simulink model "mod_sim_VTMS"  (R2018b)
settings: Solver=FixedStepDiscrete  StartTime=0.0  StopTime=t_Simulation  FixedStep=delta_t  RelTol=1e-3
values from neighbouring files (symbols this model uses):
  P_charge = 150    [main_sim_VTMS.m]
undefined symbols (not defined in the file or in its folder): A_EMaschine_Getriebe, A_j_c, A_Stirn, Anzahl_Peltierelemente, b_Batteriepack, b_c, b_EMaschine, b_Getriebe, b_j, b_Ladegeraet, BatPara, c_W, delta_t, DiscIntNeverNeededParam, e_Fahrzeug, eta_EMaschine_Break_M_EMaschine, eta_EMaschine_Break_n_EMaschine, eta_EMaschine_Faktor_Volllast, eta_EMaschine_Table, eta_Getriebe, eta_Ladegeraet, eta_Leistungselektronik_Break_M_EMaschine, eta_Leistungselektronik_Break_n_EMaschine, eta_Leistungselektronik_Faktor_Volllast, eta_Leistungselektronik_Table, f_R, I_DT_U_Break_DT, I_DT_U_Break_U, I_DT_U_Value_I, i_Getriebe, I_max, Ladevorgang, M_EMaschine_max, m_Fahrzeug, m_Zuladung, n_Zelle, P_Nebenverbraucher, p_Zelle, Peltier_Max_Eff, Q_DT_U_Break_DT, Q_DT_U_Break_U, Q_DT_U_Value_Q, Q_Imax_DT_Break_DT, Q_Imax_DT_Value_Q, r_dynamisch, rho_Luft, s_Zelle, SOC_init, Steuerung_Kuehlerluefter, Steuerung_Pumpe, Steuerung_Ventil, switch_BP_Zyklus, T_Batteriepack_init, T_EMaschine_Getriebe_init, T_Ladegeraet_init, T_Ladegeraet_Offset, T_Leistungselektronik_init, T_Offset_Batteriepack, T_Offset_EMaschine_Getriebe, T_Offset_Leistungselektronik ... (+36)
libraries: simulink x3, simulink_extras x2
(part 1 of 5)
settings Model: SimulationMode=accelerator  NumberOfSteps=100  Creator=Hannes  LastModifiedBy=gu74niw
settings SolverCC: InsertRTBMode=Always
settings DataIOCC: SaveOutput=off  SignalLogging=off  DSMLogging=off  SaveTime=off
settings OptimizationCC: DefaultParameterBehavior=Inlined  UseDivisionForNetSlopeComputation=on  PassReuseOutputArgsAs=Individual arguments  EfficientFloat2IntCast=on  EfficientMapNaN2IntZero=off  MaxStackSize=inf  SimCompilerOptimization=on
settings DebuggingCC: ReadBeforeWriteMsg=DisableAll  WriteAfterWriteMsg=DisableAll  WriteAfterReadMsg=DisableAll  AlgebraicLoopMsg=error  MultiTaskDSMMsg=none  IntegerOverflowMsg=error  ParameterUnderflowMsg=error  ParameterTunabilityLossMsg=error  AssertControl=DisableAll  AllowSymbolicDim=off  StrictBusMsg=ErrorOnBusTreatedAsVector  NonBusSignalsTreatedAsBus=error  SFInvalidInputDataAccessInChartInitDiag=error  SFTransitionOutsideNaturalParentDiag=error  SFUnreachableExecutionPathDiag=error  SFUndirectedBroadcastEventsDiag=error  SFTransitionActionBeforeConditionDiag=error  IntegerSaturationMsg=error
settings ModelReferenceCC: UpdateModelReferenceTargets=IfOutOfDate
settings SFSimCC: SFSimEcho=off  SimUseLocalCustomCode=off  MATLABDynamicMemAlloc=off
settings RTWCC: SystemTargetFile=ert.tlc  TemplateMakefile=RTW.MSVCBuild  Description=Create Visual C/C++ Solution File for Embedded Coder  GenerateReport=on  RTWUseLocalCustomCode=off  IncludeHyperlinkInReport=on  LaunchReport=on  GenerateTraceInfo=on  GenerateTraceReport=on  GenerateTraceReportSl=on  GenerateTraceReportSf=on  GenerateTraceReportEml=on
settings CodeAppCC: ForceParamTrailComments=on  IgnoreCustomStorageClasses=off  OperatorAnnotations=on  SimulinkDataObjDesc=on  SFDataObjDesc=on  InsertBlockDesc=on
settings ERTTargetCC: TargetLangStandard=C99 (ISO)  GenerateSampleERTMain=on  InlinedParameterPlacement=NonHierarchical  ERTCustomFileTemplate=example_file_process.tlc
settings ConfigComp: CovScope=ReferencedModels  CovIncludeTopModel=off

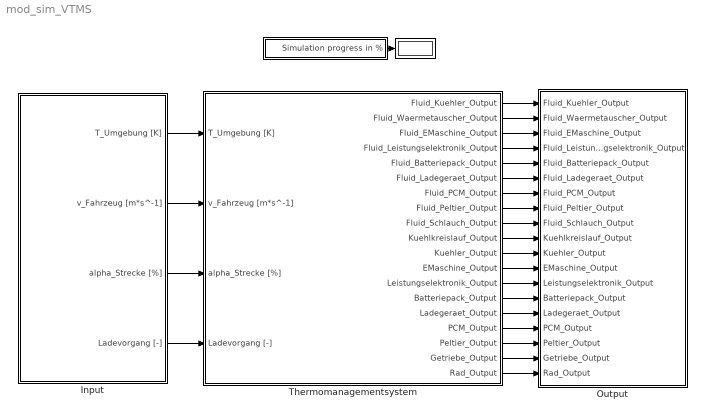
== system mod_sim_VTMS ==
  "\t\t     " : Subsystem
  " " : Display
      settings: Format=bank
  Input : Subsystem
  Output : Subsystem
  Thermomanagementsystem : Subsystem
  wires:
  "\t\t     "/1(Simulation progress in %) -> " "/1
  Input/1(T_Umgebung [K]) -> Thermomanagementsystem/1(T_Umgebung [K])
  Input/2(v_Fahrzeug [m*s^-1]) -> Thermomanagementsystem/2(v_Fahrzeug [m*s^-1])
  Input/3(alpha_Strecke [%]) -> Thermomanagementsystem/3(alpha_Strecke [%])
  Input/4(Ladevorgang [-]) -> Thermomanagementsystem/4(Ladevorgang [-])
  Thermomanagementsystem/1(Fluid_Kuehler_Output) -> Output/1(Fluid_Kuehler_Output)
  Thermomanagementsystem/2(Fluid_Waermetauscher_Output) -> Output/2(Fluid_Waermetauscher_Output)
  Thermomanagementsystem/3(Fluid_EMaschine_Output) -> Output/3(Fluid_EMaschine_Output)
  Thermomanagementsystem/4(Fluid_Leistungselektronik_Output) -> Output/4(Fluid_Leistungselektronik_Output)
  Thermomanagementsystem/5(Fluid_Batteriepack_Output) -> Output/5(Fluid_Batteriepack_Output)
  Thermomanagementsystem/6(Fluid_Ladegeraet_Output) -> Output/6(Fluid_Ladegeraet_Output)
  Thermomanagementsystem/7(Fluid_PCM_Output) -> Output/7(Fluid_PCM_Output)
  Thermomanagementsystem/8(Fluid_Peltier_Output) -> Output/8(Fluid_Peltier_Output)
  Thermomanagementsystem/9(Fluid_Schlauch_Output) -> Output/9(Fluid_Schlauch_Output)
  Thermomanagementsystem/10(Kuehlkreislauf_Output) -> Output/10(Kuehlkreislauf_Output)
  Thermomanagementsystem/11(Kuehler_Output) -> Output/11(Kuehler_Output)
  Thermomanagementsystem/12(EMaschine_Output) -> Output/12(EMaschine_Output)
  Thermomanagementsystem/13(Leistungselektronik_Output) -> Output/13(Leistungselektronik_Output)
  Thermomanagementsystem/14(Batteriepack_Output) -> Output/14(Batteriepack_Output)
  Thermomanagementsystem/15(Ladegeraet_Output) -> Output/15(Ladegeraet_Output)
  Thermomanagementsystem/16(PCM_Output) -> Output/16(PCM_Output)
  Thermomanagementsystem/17(Peltier_Output) -> Output/17(Peltier_Output)
  Thermomanagementsystem/18(Getriebe_Output) -> Output/18(Getriebe_Output)
  Thermomanagementsystem/19(Rad_Output) -> Output/19(Rad_Output)

== system mod_sim_VTMS/		      ==
  note: Fortschritt der Simulation = 100 * simulierte Zeit / t_Simulation
      |
      | mit Fortschritt der Simulation in %
  Clock : Clock
  Constant : Constant  Value=t_Simulation  VectorParams1D=off
  Divide : Product  Inputs=*/
  Umrechnung in % : Gain  Gain=100
  Simulation progress in % : Outport
  wires:
  Constant/1 -> Divide/2
  Clock/1 -> Divide/1
  Divide/1 -> Umrechnung in %/1
  Umrechnung in %/1 -> Simulation progress in %/1

== system mod_sim_VTMS/Input ==
  note: Umrechnung km/h in m/s
  note: Nur positive Geschwindigkeit
  Constant : Constant  Value=T_Umgebung
  Constant1 : Constant  Commented=on  Value=Ladevorgang
  Data Type Conversion : DataTypeConversion  OutDataTypeStr=boolean
  From Workspace : FromWorkspace  VariableName=v_Fahrzeug  SampleTime=0  OutputAfterFinalValue=Setting to zero
  From Workspace1 : FromWorkspace  VariableName=alpha_Strecke  SampleTime=0  OutputAfterFinalValue=Setting to zero
  From Workspace2 : FromWorkspace  VariableName=Ladevorgang  SampleTime=0  OutputAfterFinalValue=Setting to zero
  Gain : Gain  Gain=1/3.6
  Saturation : Saturate  UpperLimit=inf  LowerLimit=0
  T_Umgebung [K] : Outport
  v_Fahrzeug [m*s^-1] : Outport  Port=2
  alpha_Strecke [%] : Outport  Port=3
  Ladevorgang [-] : Outport  Port=4
  wires:
  Constant/1 -> T_Umgebung [K]/1
  Saturation/1 -> Gain/1
  From Workspace/1 -> Saturation/1
  Gain/1 -> v_Fahrzeug [m*s^-1]/1
  From Workspace1/1 -> alpha_Strecke [%]/1
  From Workspace2/1 -> Data Type Conversion/1
  Data Type Conversion/1 -> Ladevorgang [-]/1

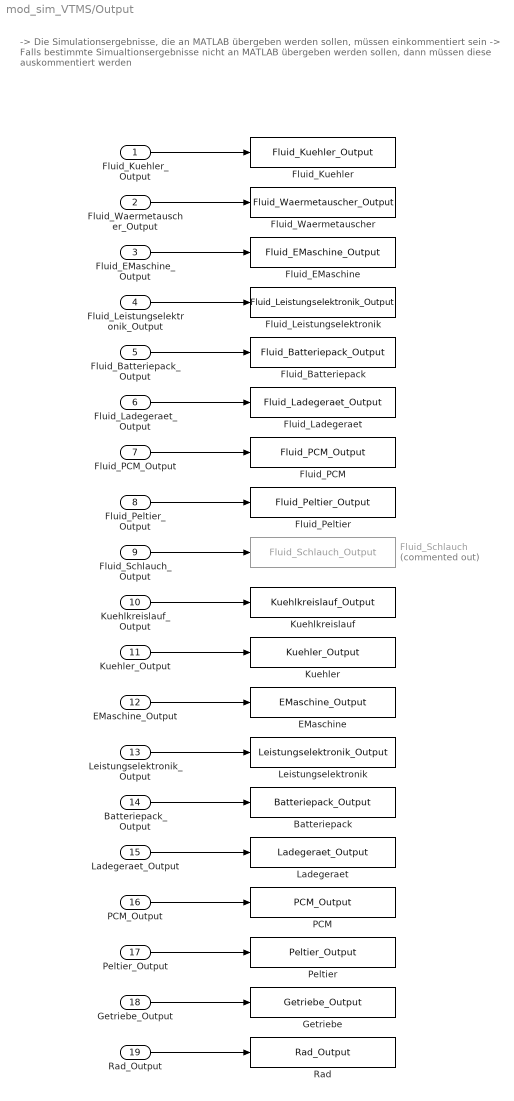
== system mod_sim_VTMS/Output ==
  note: -> Die Simulationsergebnisse, die an MATLAB übergeben werden sollen, müssen einkommentiert sein
      | -> Falls bestimmte Simualtionsergebnisse nicht an MATLAB übergeben werden sollen, dann müssen diese auskommentiert werden
  Fluid_Kuehler_Output : Inport
  Fluid_Waermetauscher_Output : Inport  Port=2
  Fluid_EMaschine_Output : Inport  Port=3
  Fluid_Leistungselektronik_Output : Inport  Port=4
  Fluid_Batteriepack_Output : Inport  Port=5
  Fluid_Ladegeraet_Output : Inport  Port=6
  Fluid_PCM_Output : Inport  Port=7
  Fluid_Peltier_Output : Inport  Port=8
  Fluid_Schlauch_Output : Inport  Port=9
  Kuehlkreislauf_Output : Inport  Port=10
  Kuehler_Output : Inport  Port=11
  EMaschine_Output : Inport  Port=12
  Leistungselektronik_Output : Inport  Port=13
  Batteriepack_Output : Inport  Port=14
  Ladegeraet_Output : Inport  Port=15
  PCM_Output : Inport  Port=16
  Peltier_Output : Inport  Port=17
  Getriebe_Output : Inport  Port=18
  Rad_Output : Inport  Port=19
  Batteriepack : ToWorkspace  VariableName=Batteriepack_Output  SaveFormat=Timeseries  SampleTime=-1
      settings: Decimation=Decimation_Output
  EMaschine : ToWorkspace  VariableName=EMaschine_Output  SaveFormat=Timeseries  SampleTime=-1
      settings: Decimation=Decimation_Output
  Fluid_Batteriepack : ToWorkspace  VariableName=Fluid_Batteriepack_Output  SaveFormat=Timeseries  SampleTime=-1
      settings: Decimation=Decimation_Output
  Fluid_EMaschine : ToWorkspace  VariableName=Fluid_EMaschine_Output  SaveFormat=Timeseries  SampleTime=-1
      settings: Decimation=Decimation_Output
  Fluid_Kuehler : ToWorkspace  VariableName=Fluid_Kuehler_Output  SaveFormat=Timeseries  SampleTime=-1
      settings: Decimation=Decimation_Output
  Fluid_Ladegeraet : ToWorkspace  VariableName=Fluid_Ladegeraet_Output  SaveFormat=Timeseries  SampleTime=-1
      settings: Decimation=Decimation_Output
  Fluid_Leistungselektronik : ToWorkspace  VariableName=Fluid_Leistungselektronik_Output  SaveFormat=Timeseries  SampleTime=-1
      settings: Decimation=Decimation_Output
  Fluid_PCM : ToWorkspace  VariableName=Fluid_PCM_Output  SaveFormat=Timeseries  SampleTime=-1
      settings: Decimation=Decimation_Output
  Fluid_Peltier : ToWorkspace  VariableName=Fluid_Peltier_Output  SaveFormat=Timeseries  SampleTime=-1
      settings: Decimation=Decimation_Output
  Fluid_Schlauch : ToWorkspace  Commented=on  VariableName=Fluid_Schlauch_Output  SaveFormat=Timeseries  SampleTime=-1
      settings: Decimation=Decimation_Output
  Fluid_Waermetauscher : ToWorkspace  VariableName=Fluid_Waermetauscher_Output  SaveFormat=Timeseries  SampleTime=-1
      settings: Decimation=Decimation_Output
  Getriebe : ToWorkspace  VariableName=Getriebe_Output  SaveFormat=Timeseries  SampleTime=-1
      settings: Decimation=Decimation_Output
  Kuehler : ToWorkspace  VariableName=Kuehler_Output  SaveFormat=Timeseries  SampleTime=-1
      settings: Decimation=Decimation_Output
  Kuehlkreislauf : ToWorkspace  VariableName=Kuehlkreislauf_Output  SaveFormat=Timeseries  SampleTime=-1
      settings: Decimation=Decimation_Output
  Ladegeraet : ToWorkspace  VariableName=Ladegeraet_Output  SaveFormat=Timeseries  SampleTime=-1
      settings: Decimation=Decimation_Output
  Leistungselektronik : ToWorkspace  VariableName=Leistungselektronik_Output  SaveFormat=Timeseries  SampleTime=-1
      settings: Decimation=Decimation_Output
  PCM : ToWorkspace  VariableName=PCM_Output  SaveFormat=Timeseries  SampleTime=-1
      settings: Decimation=Decimation_Output
  Peltier : ToWorkspace  VariableName=Peltier_Output  SaveFormat=Timeseries  SampleTime=-1
      settings: Decimation=Decimation_Output
  Rad : ToWorkspace  VariableName=Rad_Output  SaveFormat=Timeseries  SampleTime=-1
      settings: Decimation=Decimation_Output
  wires:
  Ladegeraet_Output/1 -> Ladegeraet/1
  Fluid_Ladegeraet_Output/1 -> Fluid_Ladegeraet/1
  PCM_Output/1 -> PCM/1
  Kuehler_Output/1 -> Kuehler/1
  Kuehlkreislauf_Output/1 -> Kuehlkreislauf/1
  Fluid_PCM_Output/1 -> Fluid_PCM/1
  Fluid_Kuehler_Output/1 -> Fluid_Kuehler/1
  Fluid_EMaschine_Output/1 -> Fluid_EMaschine/1
  Leistungselektronik_Output/1 -> Leistungselektronik/1
  Rad_Output/1 -> Rad/1
  Fluid_Schlauch_Output/1 -> Fluid_Schlauch/1
  Fluid_Peltier_Output/1 -> Fluid_Peltier/1
  EMaschine_Output/1 -> EMaschine/1
  Fluid_Batteriepack_Output/1 -> Fluid_Batteriepack/1
  Fluid_Leistungselektronik_Output/1 -> Fluid_Leistungselektronik/1
  Batteriepack_Output/1 -> Batteriepack/1
  Getriebe_Output/1 -> Getriebe/1
  Peltier_Output/1 -> Peltier/1
  Fluid_Waermetauscher_Output/1 -> Fluid_Waermetauscher/1

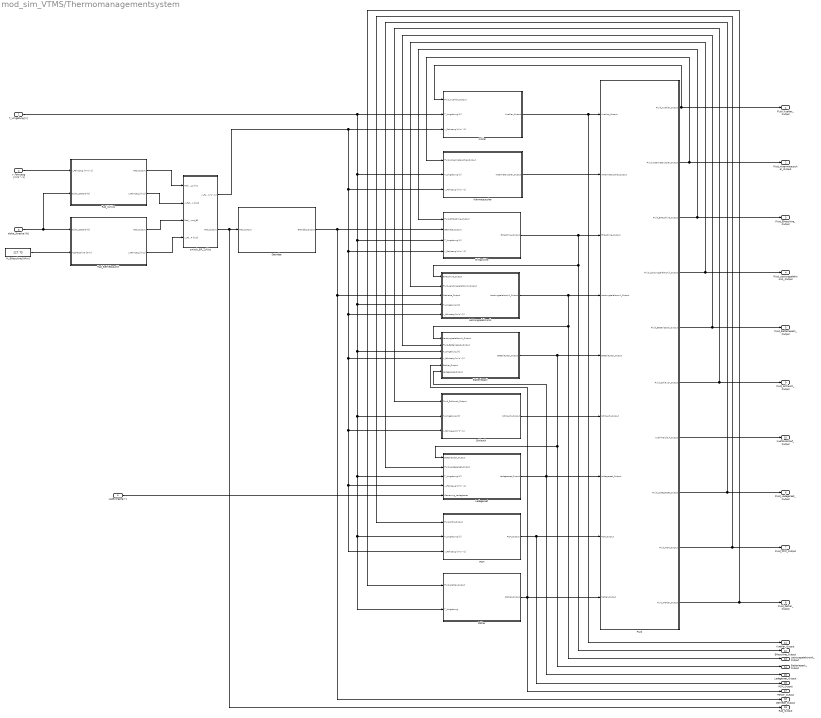
== system mod_sim_VTMS/Thermomanagementsystem ==
  T_Umgebung [K] : Inport
  v_Fahrzeug [m*s^-1] : Inport  Port=2
  alpha_Strecke [%] : Inport  Port=3
  Ladevorgang [-] : Inport  Port=4
  Batteriepack : Subsystem
  E-Maschine : Subsystem
  Fluid : Subsystem
  Getriebe : Subsystem
  Kühler : Subsystem
  Ladegeraet : Subsystem
  Leistungselektronik : Subsystem
  M_EMaschine [N*m] : Constant  Value=127.75
  PCM : Subsystem
  Peltier : Subsystem
  Rad_Betriebspunkt : Subsystem
  Rad_Zyklus : Subsystem
  Schlauch : Subsystem
  Wärmetauscher : Subsystem
  switch_BP_Zyklus : Subsystem
  Fluid_Kuehler_Output : Outport
  Fluid_Waermetauscher_Output : Outport  Port=2
  Fluid_EMaschine_Output : Outport  Port=3
  Fluid_Leistungselektronik_Output : Outport  Port=4
  Fluid_Batteriepack_Output : Outport  Port=5
  Fluid_Ladegeraet_Output : Outport  Port=6
  Fluid_PCM_Output : Outport  Port=7
  Fluid_Peltier_Output : Outport  Port=8
  Fluid_Schlauch_Output : Outport  Port=9
  Kuehlkreislauf_Output : Outport  Port=10
  Kuehler_Output : Outport  Port=11
  EMaschine_Output : Outport  Port=12
  Leistungselektronik_Output : Outport  Port=13
  Batteriepack_Output : Outport  Port=14
  Ladegeraet_Output : Outport  Port=15
  PCM_Output : Outport  Port=16
  Peltier_Output : Outport  Port=17
  Getriebe_Output : Outport  Port=18
  Rad_Output : Outport  Port=19
  wires:
  alpha_Strecke [%]/1 -> Rad_Zyklus/2(alpha_Strecke [%]), Rad_Betriebspunkt/1(alpha_Strecke [%])
  Getriebe/1(Getriebe_Output) -> E-Maschine/2(Getriebe_Output), Getriebe_Output/1, Leistungselektronik/3(Getriebe_Output)
  E-Maschine/1(EMaschine_Output) -> Leistungselektronik/1(EMaschine_Output), EMaschine_Output/1, Fluid/3(EMaschine_Output)
  Leistungselektronik/1(Leistungselektronik_Output) -> Batteriepack/1(Leistungselektronik_Output), Leistungselektronik_Output/1, Fluid/4(Leistungselektronik_Output)
  Batteriepack/1(Batteriepack_Output) -> Fluid/5(Batteriepack_Output), Ladegeraet/1(Batteriepack_Output), Batteriepack_Output/1
  Fluid/6(Fluid_Schlauch_Output) -> Fluid_Schlauch_Output/1, Schlauch/1(Fluid_Schlauch_Output)
  Wärmetauscher/1(Waermetauscher_Output) -> Fluid/2(Waermetauscher_Output)
  T_Umgebung [K]/1 -> Kühler/2(T_Umgebung [K]), Ladegeraet/3(T_Umgebung [K]), Peltier/2(T_Umgebung), PCM/2(T_Umgebung [K]), Schlauch/2(T_Umgebung [K]), Batteriepack/3(T_Umgebung [K]), Leistungselektronik/4(T_Umgebung [K]), E-Maschine/3(T_Umgebung [K]), Wärmetauscher/2(T_Umgebung [K])
  Kühler/1(Kuehler_Output) -> Kuehler_Output/1, Fluid/1(Kuehler_Output)
  Fluid/2(Fluid_Waermetauscher_Output) -> Fluid_Waermetauscher_Output/1, Wärmetauscher/1(Fluid_Waermetauscher_Output)
  Fluid/4(Fluid_Leistungselektronik_Output) -> Fluid_Leistungselektronik_Output/1, Leistungselektronik/2(Fluid_Leistungselektronik_Output)
  Fluid/5(Fluid_Batteriepack_Output) -> Fluid_Batteriepack_Output/1, Batteriepack/2(Fluid_Batteriepack_Output)
  Schlauch/1(Schlauch_Output) -> Fluid/6(Schlauch_Output)
  Fluid/1(Fluid_Kuehler_Output) -> Fluid_Kuehler_Output/1, Kühler/1(Fluid_Kuehler_Output)
  Fluid/3(Fluid_EMaschine_Output) -> Fluid_EMaschine_Output/1, E-Maschine/1(Fluid_EMaschine_Output)
  Fluid/7(Kuehlkreislauf_Output) -> Kuehlkreislauf_Output/1
  Ladegeraet/1(Ladegeraet_Output) -> Ladegeraet_Output/1, Batteriepack/6(Ladegeraet_Output), Fluid/7(Ladegeraet_Output)
  PCM/1(PCM_Output) -> PCM_Output/1, Fluid/8(PCM_Output)
  Ladevorgang [-]/1 -> Ladegeraet/5(Steuerung_Ladegeraet)
  Peltier/1(Peltier_Output) -> Peltier_Output/1, Batteriepack/5(Peltier_Output), Fluid/9(Peltier_Output)
  Fluid/8(Fluid_Ladegeraet_Output) -> Ladegeraet/2(Fluid_Ladegeraet_Output), Fluid_Ladegeraet_Output/1
  Fluid/9(Fluid_PCM_Output) -> Fluid_PCM_Output/1, PCM/1(Fluid_PCM_Output)
  Fluid/10(Fluid_Peltier_Output) -> Peltier/1(Fluid_Peltier_Output), Fluid_Peltier_Output/1
  M_EMaschine [N*m]/1 -> Rad_Betriebspunkt/2(M_EMaschine [N*m])
  v_Fahrzeug [m*s^-1]/1 -> Rad_Zyklus/1(v_Fahrzeug [m*s^-1])
  switch_BP_Zyklus/1(v_Fahrzeug [m*s^-1]) -> Kühler/3(v_Fahrzeug [m*s^-1]), Ladegeraet/4(v_Fahrzeug [m*s^-1]), PCM/3(v_Fahrzeug [m*s^-1]), Schlauch/3(v_Fahrzeug [m*s^-1]), Batteriepack/4(v_Fahrzeug [m*s^-1]), Leistungselektronik/5(v_Fahrzeug [m*s^-1]), E-Maschine/4(v_Fahrzeug [m*s^-1]), Wärmetauscher/3(v_Fahrzeug [m*s^-1])
  switch_BP_Zyklus/2(Rad_Output) -> Rad_Output/1, Getriebe/1(Rad_Output)
  Rad_Zyklus/1(Rad_Output) -> switch_BP_Zyklus/1(Rad_Output_Zyklus)
  Rad_Zyklus/2(v_Fahrzeug [m/s]) -> switch_BP_Zyklus/2(v_Fahrzeug_Zyklus [m/s])
  Rad_Betriebspunkt/1(Rad_Output) -> switch_BP_Zyklus/3(Rad_Output_BP)
  Rad_Betriebspunkt/2(v_Fahrzeug [m/s]) -> switch_BP_Zyklus/4(v_Fahrzeug_BP [m/s])

== system mod_sim_VTMS/Thermomanagementsystem/Batteriepack ==
  note: Neben der Leistungsanforderung aus dem Fahrbetrieb belasten Nebenverbraucher des Fahrzeugs das Batteriepack
  Leistungselektronik_Output : Inport
  Fluid_Batteriepack_Output : Inport  Port=2
  T_Umgebung [K] : Inport  Port=3
  v_Fahrzeug [m*s^-1] : Inport  Port=4
  Peltier_Output : Inport  Port=5
  Ladegeraet_Output : Inport  Port=6
  "Abbruch, wenn SOC <= 0" : Subsystem
  Add : Sum  Inputs=++-+
  Batteriepack(1) elektrisch : Subsystem
  Batteriepack(1) thermisch : Subsystem
  Bus Creator : BusCreator  Inputs=6
  Bus Selector : BusSelector  OutputSignals=T_FinitesVolumen_Batteriepack(1) [K],PV_Kuehlfluessigkeit_Batteriepack(1) [m^3*s^-1]
  Bus Selector1 : BusSelector  OutputSignals=P_Batteriepack_Fahrbetrieb [W]
  Bus Selector2 : BusSelector  OutputSignals=P_Ladegeraet_Bat [W]
  Bus Selector3 : BusSelector  OutputSignals=P_Peltier_Bat [W]
  Constant : Constant  Value=P_Nebenverbraucher  VectorParams1D=off
  Batteriepack_Output : Outport
  wires:
  Bus Creator/1 -> Batteriepack_Output/1
  Batteriepack(1) elektrisch/5(P_Verlust_Batteriepack [W]) -> Batteriepack(1) thermisch/1(P_Verlust_Batteriepack [W])
  T_Umgebung [K]/1 -> Batteriepack(1) thermisch/4(T_Umgebung [K])
  v_Fahrzeug [m*s^-1]/1 -> Batteriepack(1) thermisch/5(v_Fahrzeug [m*s^-1])
  Batteriepack(1) thermisch/1(T_Batteriepack [K]) -> Batteriepack(1) elektrisch/1(T_Batteriepack [K]), Bus Creator/5  "T_Batteriepack [K]"
  Batteriepack(1) elektrisch/4(eta_Batteriepack [%]) -> Bus Creator/4  "eta_Batteriepack [%]"
  Batteriepack(1) elektrisch/2(U_Batteriepack [V]) -> Bus Creator/2  "U_Batteriepack [V]"
  Batteriepack(1) elektrisch/1(I_Batteriepack [A]) -> Bus Creator/1  "I_Batteriepack [A]"
  Batteriepack(1) thermisch/2(PQ_Batteriepack_FinitesVolumen [W]) -> Bus Creator/6  "PQ_Batteriepack(1)_FinitesVolumen [W]"
  Batteriepack(1) elektrisch/3(SOC_Batteriepack [-]) -> "Abbruch, wenn SOC <= 0"/1(SOC_Batteriepack [-]), Bus Creator/3  "SOC_Batteriepack [-]"
  Fluid_Batteriepack_Output/1 -> Bus Selector/1
  Bus Selector/1 -> Batteriepack(1) thermisch/2(T_FinitesVolumen [K])  "<T_FinitesVolumen_Batteriepack(1) [K]>"
  Bus Selector/2 -> Batteriepack(1) thermisch/3(PV_Kuehlfluessigkeit [m^3*s^-1])  "<PV_Kuehlfluessigkeit_Batteriepack(1) [m^3*s^-1]>"
  Bus Selector3/1 -> Add/4  "<P_Peltier_Bat [W]>"
  Bus Selector2/1 -> Add/3  "<P_Ladegeraet_Bat [W]>"
  Ladegeraet_Output/1 -> Bus Selector2/1
  Bus Selector1/1 -> Add/1  "<P_Batteriepack_Fahrbetrieb [W]>"
  Constant/1 -> Add/2
  Add/1 -> Batteriepack(1) elektrisch/2(P_Batteriepack [W])
  Peltier_Output/1 -> Bus Selector3/1
  Leistungselektronik_Output/1 -> Bus Selector1/1

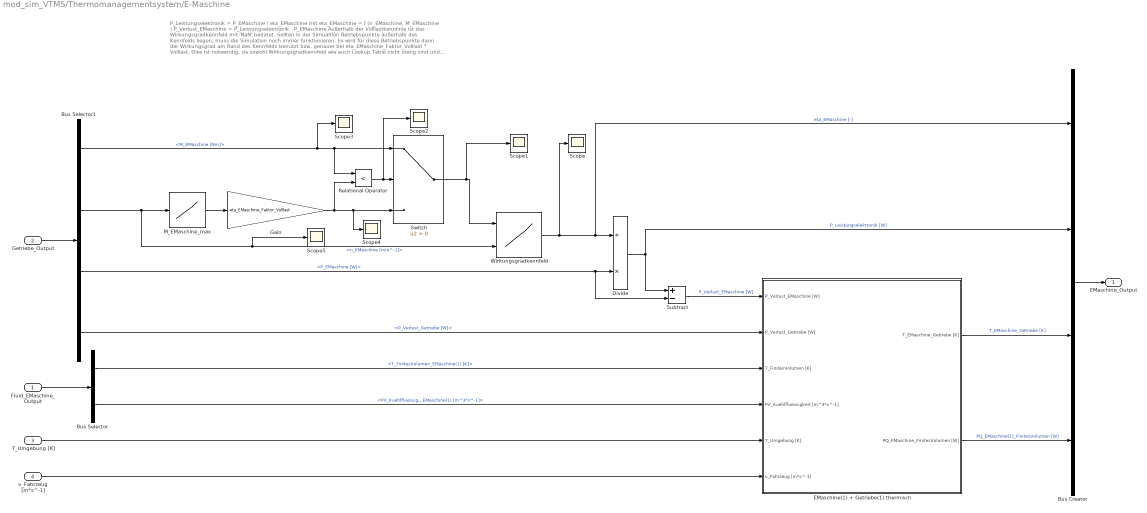
== system mod_sim_VTMS/Thermomanagementsystem/E-Maschine ==
  note: P_Leistungselektronik = P_EMaschine / eta_EMaschine
      |
      | mit eta_EMaschine = f (n_EMaschine, M_EMaschine )
      |
      | P_Verlust_EMaschine = P_Leistungselektronik - P_EMaschine
      |
      | Außerhalb der Volllastkennlinie ist das Wirkungsgradkennfeld mit 'NaN' bedatet. Sollten in der Simualtion Betriebspunkte außerhalb des Kennfelds liegen, muss die Simulation noch immer funktionieren. Es wird für diese Betriebspunkte dann der Wirkungsgrad am Rand des Kennfelds benutzt bzw. genauer bei eta_EMaschine_Faktor_Volllast * Volllast. Dies ist notwendig, da sowohl Wirkungsgradkennfeld wie auch Lookup Table nicht stetig sind und somit zwischen Stützstellen interpolieren müssen. Dies kann dazu führen, dass ein Wert, der auf der Volllastlinie sitzt, in 'NaN' im Wirkungsgradkennfeld resultiert. Um dies zu vermeiden, wird mit eta_EMaschine_Faktor_Volllast * Volllast gerechnet, wenn Betriebspunkte außerhalb des Kennfelds liegen, um 'NaN' Wirkungsgrade zu vermeiden. eta_EMaschine_Faktor_Volllast ist stark abh. von der Güte (Abstand der Stützstellen) des Wirkungsgradkennfeldes.
  Fluid_EMaschine_Output : Inport
  Getriebe_Output : Inport  Port=2
  T_Umgebung [K] : Inport  Port=3
  v_Fahrzeug [m*s^-1] : Inport  Port=4
  Bus Creator : BusCreator  Inputs=4
  Bus Selector : BusSelector  OutputSignals=T_FinitesVolumen_EMaschine(1) [K],PV_Kuehlfluessigkeit_EMaschine(1) [m^3*s^-1]
  Bus Selector1 : BusSelector  OutputSignals=M_EMaschine [Nm],n_EMaschine [min^-1],P_EMaschine [W],P_Verlust_Getriebe [W]
  Divide : Product  Inputs=/*
  EMaschine(1) + Getriebe(1) thermisch : Subsystem
  Gain : Gain  Gain=eta_EMaschine_Faktor_Volllast
  M_EMaschine_max : Lookup_n-D  NumberOfTableDimensions=1  BreakpointsForDimension1=M_EMaschine_max(1,:)  BeginIndexSearchUsingPreviousIndexResult=on  Table=M_EMaschine_max(2,:)  ExtrapMethod=Clip  UseLastTableValue=on  InternalRulePriority=Speed  RndMeth=Simplest  InputSameDT=on
  Relational Operator : RelationalOperator  Operator=<  OutDataTypeStr=boolean  RndMeth=Simplest
  Scope{,1..5} (6 alike) : Scope
  Subtract : Sum  Inputs=+-
  Switch : Switch  Criteria=u2 > Threshold
  Wirkungsgradkennfeld : Lookup_n-D  BreakpointsForDimension1=eta_EMaschine_Break_M_EMaschine  BreakpointsForDimension2=eta_EMaschine_Break_n_EMaschine  BeginIndexSearchUsingPreviousIndexResult=on  Table=eta_EMaschine_Table  ExtrapMethod=Clip  UseLastTableValue=on  InternalRulePriority=Speed  RndMeth=Simplest  InputSameDT=on
  EMaschine_Output : Outport
  wires:
  Bus Selector1/2 -> Scope5/1, Wirkungsgradkennfeld/2, M_EMaschine_max/1  "<n_EMaschine [min^-1]>"
  Getriebe_Output/1 -> Bus Selector1/1
  Bus Selector1/1 -> Scope3/1, Relational Operator/1, Switch/1  "<M_EMaschine [Nm]>"
  Bus Creator/1 -> EMaschine_Output/1
  EMaschine(1) + Getriebe(1) thermisch/2(PQ_EMaschine_FinitesVolumen [W]) -> Bus Creator/4  "PQ_EMaschine(1)_FinitesVolumen [W]"
  EMaschine(1) + Getriebe(1) thermisch/1(T_EMaschine_Getriebe [K]) -> Bus Creator/3  "T_EMaschine_Getriebe [K]"
  Bus Selector1/3 -> Subtract/2, Divide/2  "<P_EMaschine [W]>"
  Divide/1 -> Subtract/1, Bus Creator/2  "P_Leistungselektronik [W]"
  T_Umgebung [K]/1 -> EMaschine(1) + Getriebe(1) thermisch/5(T_Umgebung [K])
  Subtract/1 -> EMaschine(1) + Getriebe(1) thermisch/1(P_Verlust_EMaschine [W])  "P_Verlust_EMaschine [W]"
  Wirkungsgradkennfeld/1 -> Scope/1, Bus Creator/1, Divide/1  "eta_EMaschine [-]"
  Relational Operator/1 -> Scope2/1, Switch/2
  M_EMaschine_max/1 -> Gain/1
  Switch/1 -> Scope1/1, Wirkungsgradkennfeld/1
  Gain/1 -> Relational Operator/2, Scope4/1, Switch/3
  Bus Selector1/4 -> EMaschine(1) + Getriebe(1) thermisch/2(P_Verlust_Getriebe [W])  "<P_Verlust_Getriebe [W]>"
  v_Fahrzeug [m*s^-1]/1 -> EMaschine(1) + Getriebe(1) thermisch/6(v_Fahrzeug [m*s^-1])
  Fluid_EMaschine_Output/1 -> Bus Selector/1
  Bus Selector/2 -> EMaschine(1) + Getriebe(1) thermisch/4(PV_Kuehlfluessigkeit [m^3*s^-1])  "<PV_Kuehlfluessigkeit_EMaschine(1) [m^3*s^-1]>"
  Bus Selector/1 -> EMaschine(1) + Getriebe(1) thermisch/3(T_FinitesVolumen [K])  "<T_FinitesVolumen_EMaschine(1) [K]>"

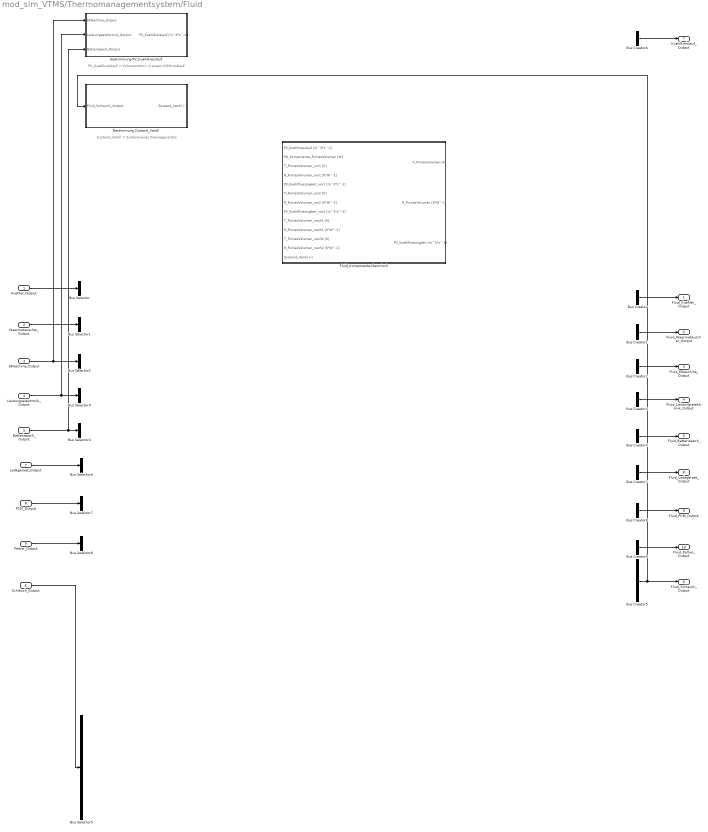
== system mod_sim_VTMS/Thermomanagementsystem/Fluid ==
  note: PV_Kuehlkreislauf = Volumenstrom in einem Kühlkreislauf
  note: Zustand_Ventil = Zustand eines Dreiwegeventils
  Kuehler_Output : Inport
  Waermetauscher_Output : Inport  Port=2
  EMaschine_Output : Inport  Port=3
  Leistungselektronik_Output : Inport  Port=4
  Batteriepack_Output : Inport  Port=5
  Schlauch_Output : Inport  Port=6
  Ladegeraet_Output : Inport  Port=7
  PCM_Output : Inport  Port=8
  Peltier_Output : Inport  Port=9
  Bestimmung PV_Kuehlkreislauf : Subsystem
  Bestimmung Zustand_Ventil : Subsystem
  Bus Creator{,2..4,6..7,9} (7 alike) : BusCreator  Inputs=2
  Bus Creator1 : BusCreator  Inputs=4
  Bus Creator5 : BusCreator  Inputs=22
  Bus Creator8 : BusCreator  Inputs=4
  Bus Selector : BusSelector  OutputSignals=PQ_Kuehler(1)_FinitesVolumen [W]
  Bus Selector1 : BusSelector  OutputSignals=PQ_Waermetauscher(1_1)_FinitesVolumen [W],PQ_Waermetauscher(2_1)_FinitesVolumen [W]
  Bus Selector2 : BusSelector  OutputSignals=PQ_EMaschine(1)_FinitesVolumen [W]
  Bus Selector3 : BusSelector  OutputSignals=PQ_Leistungselektronik(1)_FinitesVolumen [W]
  Bus Selector4 : BusSelector  OutputSignals=PQ_Batteriepack(1)_FinitesVolumen [W]
  Bus Selector5 : BusSelector  OutputSignals=PQ_Schlauch(1)_FinitesVolumen [W],PQ_Schlauch(2)_FinitesVolumen [W],PQ_Schlauch(3)_FinitesVolumen [W],PQ_Schlauch(4)_FinitesVolumen [W],PQ_Schlauch(5)_FinitesVolumen [W],PQ_Schlauch(6)_FinitesVolumen [W],PQ_Schlauch(7)_FinitesVolumen [W],PQ_Schlauch(8)_FinitesVolumen [W],PQ_Schlauch(9)_FinitesVolumen [W],PQ_Schlauch(10)_FinitesVolumen [W],PQ_Schlauch(11)_FinitesVolumen [W]
  Bus Selector6 : BusSelector  OutputSignals=PQ_Ladegeraet(1)_FinitesVolumen [W]
  Bus Selector7 : BusSelector  OutputSignals=PQ_PCM(1)_FinitesVolumen [W],PQ_PCM(2)_FinitesVolumen [W]
  Bus Selector8 : BusSelector  OutputSignals=PQ_Peltier(1)_FinitesVolumen [W]
  Fluid_Komponente thermisch : Subsystem
  Fluid_Kuehler_Output : Outport
  Fluid_Waermetauscher_Output : Outport  Port=2
  Fluid_EMaschine_Output : Outport  Port=3
  Fluid_Leistungselektronik_Output : Outport  Port=4
  Fluid_Batteriepack_Output : Outport  Port=5
  Fluid_Schlauch_Output : Outport  Port=6  OutDataTypeStr=double
  Kuehlkreislauf_Output : Outport  Port=7
  Fluid_Ladegeraet_Output : Outport  Port=8
  Fluid_PCM_Output : Outport  Port=9
  Fluid_Peltier_Output : Outport  Port=10
  wires:
  Bus Creator4/1 -> Fluid_Batteriepack_Output/1
  Bus Creator3/1 -> Fluid_Leistungselektronik_Output/1
  Bus Creator2/1 -> Fluid_EMaschine_Output/1
  Bus Creator1/1 -> Fluid_Waermetauscher_Output/1
  Bus Creator5/1 -> Fluid_Schlauch_Output/1, Bestimmung Zustand_Ventil/1(Fluid_Schlauch_Output)
  Bus Creator/1 -> Fluid_Kuehler_Output/1
  Schlauch_Output/1 -> Bus Selector5/1
  Batteriepack_Output/1 -> Bestimmung PV_Kuehlkreislauf/3(Batteriepack_Output), Bus Selector4/1
  Leistungselektronik_Output/1 -> Bestimmung PV_Kuehlkreislauf/2(Leistungselektronik_Output), Bus Selector3/1
  EMaschine_Output/1 -> Bestimmung PV_Kuehlkreislauf/1(EMaschine_Output), Bus Selector2/1
  Waermetauscher_Output/1 -> Bus Selector1/1
  Kuehler_Output/1 -> Bus Selector/1
  Bus Creator6/1 -> Kuehlkreislauf_Output/1
  Ladegeraet_Output/1 -> Bus Selector6/1
  PCM_Output/1 -> Bus Selector7/1
  Peltier_Output/1 -> Bus Selector8/1
  Bus Creator7/1 -> Fluid_Ladegeraet_Output/1
  Bus Creator8/1 -> Fluid_PCM_Output/1
  Bus Creator9/1 -> Fluid_Peltier_Output/1

== system mod_sim_VTMS/Thermomanagementsystem/Getriebe ==
  note: -> Mit dieser Version des Thermomanagementsystemmodells ist keine Rekuperation simulierbar
      | -> Annahme: Bremsmomente werden komplett von der Reibungsbremse abgefangen
      | -> Deswegen werden von den Rädern an das Getriebe und an die E-Maschine nur positive und keine negativen Drehmomente und Leistungsanforderungen übertragen (Blöcke "Saturation")
      | -> Deswegen werden von den Rädern an den gesamten Antriebsstrang (Getriebe, E-Maschine, Leistungselektronik und Batteriepack) nur positive und keine negativen Leistungsanforderungen übertragen
      |
      | n_EMaschine = n_Rad * i_Getriebe
      |
      | M_EMaschine = M_Rad / (i_Getriebe * eta_Getriebe)
      |
      | P_EMaschine = P_Rad / eta_Getriebe
      |
      | P_Verlust_Getriebe = P_EMaschine - P_Rad
  Rad_Output : Inport
  Bus Creator : BusCreator  Inputs=4
  Bus Selector : BusSelector  OutputSignals=n_Rad [min^-1],M_Rad [Nm],P_Rad [W]
  Constant : Constant  Value=i_Getriebe
  Constant1 : Constant  Value=eta_Getriebe
  Divide : Product  Inputs=/*/
  Divide1 : Product  Inputs=/*
  Product : Product
  Saturation : Saturate  UpperLimit=inf  LowerLimit=0
  Saturation1 : Saturate  UpperLimit=inf  LowerLimit=0
  Subtract : Sum  Inputs=+-
  Getriebe_Output : Outport
  wires:
  Bus Creator/1 -> Getriebe_Output/1
  Rad_Output/1 -> Bus Selector/1
  Constant/1 -> Divide/1, Product/2
  Bus Selector/2 -> Saturation/1  "<M_Rad [Nm]>"
  Divide/1 -> Bus Creator/2  "M_EMaschine [Nm]"
  Bus Selector/1 -> Product/1  "<n_Rad [min^-1]>"
  Product/1 -> Bus Creator/1  "n_EMaschine [min^-1]"
  Constant1/1 -> Divide1/1, Divide/3
  Bus Selector/3 -> Saturation1/1  "<P_Rad [W]>"
  Divide1/1 -> Subtract/1, Bus Creator/3  "P_EMaschine [W]"
  Saturation/1 -> Divide/2
  Saturation1/1 -> Subtract/2, Divide1/2
  Subtract/1 -> Bus Creator/4  "P_Verlust_Getriebe [W]"

== system mod_sim_VTMS/Thermomanagementsystem/Kühler ==
  Fluid_Kuehler_Output : Inport
  T_Umgebung [K] : Inport  Port=2
  v_Fahrzeug [m*s^-1] : Inport  Port=3
  Bus Creator : BusCreator  Inputs=2
  Bus Selector : BusSelector  OutputSignals=T_FinitesVolumen_Kuehler(1) [K],PV_Kuehlfluessigkeit_Kuehler(1) [m^3*s^-1]
  Kuehler thermisch : Subsystem
  Kuehler_Output : Outport
  wires:
  Bus Creator/1 -> Kuehler_Output/1
  Fluid_Kuehler_Output/1 -> Bus Selector/1

== system mod_sim_VTMS/Thermomanagementsystem/Ladegeraet ==
  note: Der Ladevorgang kann simuliert werden.
      | Wärend des Ladevorgangs führt eine Verlustleistung zum Aufheizen des Ladegeräts.
      | Die Ladeleistung wird an das Batteriepack weitergeleitet und führt zu einem Ansteig des SOC.
      | Das Ladegerät hat eine Masse und folglich eine Temperatur. Während der Fahrt fungiert es als thermische Masse und kann folglich Wärme mit dem Kühlkreislaufsystem austauschen.
  Batteriepack_Output : Inport
  Fluid_Ladegeraet_Output : Inport  Port=2
  T_Umgebung [K] : Inport  Port=3
  v_Fahrzeug [m*s^-1] : Inport  Port=4
  Steuerung_Ladegeraet : Inport  Port=5
  Bus Creator : BusCreator  Inputs=3
  Bus Selector : BusSelector  OutputSignals=T_FinitesVolumen_Ladegeraet(1) [K],PV_Kuehlfluessigkeit_Ladegeraet(1) [m^3*s^-1]
  Delay : Delay  DelayLength=1  InitialCondition=0
  Ladegeraet(1) elektrisch : Subsystem
  Ladegeraet(1) thermisch : Subsystem
  Ladegeraet_Output : Outport
  wires:
  Bus Creator/1 -> Ladegeraet_Output/1
  T_Umgebung [K]/1 -> Ladegeraet(1) thermisch/4(T_Umgebung [K])
  v_Fahrzeug [m*s^-1]/1 -> Ladegeraet(1) thermisch/5(v_Fahrzeug [m*s^-1])
  Ladegeraet(1) thermisch/1(T_Ladegeraet [K]) -> Bus Creator/2  "T_Ladegeraet [K]"
  Ladegeraet(1) thermisch/2(PQ_Ladegeraet_FinitesVolumen [W]) -> Bus Creator/3  "PQ_Ladegeraet(1)_FinitesVolumen [W]"
  Fluid_Ladegeraet_Output/1 -> Bus Selector/1
  Bus Selector/1 -> Ladegeraet(1) thermisch/2(T_FinitesVolumen [K])  "<T_FinitesVolumen_Ladegeraet(1) [K]>"
  Bus Selector/2 -> Ladegeraet(1) thermisch/3(PV_Kuehlfluessigkeit [m^3*s^-1])  "<PV_Kuehlfluessigkeit_Ladegeraet(1) [m^3*s^-1]>"
  Ladegeraet(1) elektrisch/2(Verlustleistung_Ladegeraet [W]) -> Ladegeraet(1) thermisch/1(P_Verlust_Ladegeraet [W])  "Verlustleistung_Ladegeraet [W]"
  Batteriepack_Output/1 -> Ladegeraet(1) elektrisch/1(Batteriepack_Output)
  Ladegeraet(1) elektrisch/1(Leistung_Ladegeraet_Bat [W]) -> Delay/1  "P_Ladegeraet_Bat [W]"
  Steuerung_Ladegeraet/1 -> Ladegeraet(1) elektrisch/2(Steuerungssignal)
  Delay/1 -> Bus Creator/1  "P_Ladegeraet_Bat [W]"

== system mod_sim_VTMS/Thermomanagementsystem/Leistungselektronik ==
  note: P_Batteriepack_Fahrbetrieb = P_Leistungselektronik / eta_Leistungselektronik
      |
      | mit eta_Leistungselektronik = f (n_EMaschine,M_EMaschine)
      |
      | P_Verlust_Leistungselektronik = P_Batteriepack_Fahrbetrieb - P_Leistungselektronik
      |
      | Außerhalb der Volllastkennlinie ist das Wirkungsgradkennfeld mit 'NaN' bedatet. Sollten in der Simualtion Betriebspunkte außerhalb des Kennfelds liegen, muss die Simulation noch immer funktionieren. Es wird für diese Betriebspunkte dann der Wirkungsgrad am Rand des Kennfelds benutzt bzw. genauer bei eta_Leistungselektronik_Faktor_Volllast * Volllast. Dies ist notwendig, da sowohl Wirkungsgradkennfeld wie auch Lookup Table nicht stetig sind und somit zwischen Stützstellen interpolieren müssen. Dies kann dazu führen, dass ein Wert, der auf der Volllastlinie sitzt, in 'NaN' im Wirkungsgradkennfeld resultiert. Um dies zu vermeiden, wird mit eta_Leistungselektronik_Faktor_Volllast * Volllast gerechnet, wenn Betriebspunkte außerhalb des Kennfelds liegen, um 'NaN' Wirkungsgrade zu vermeiden. eta_Leistungselektronik_Faktor_Volllast ist stark abh. von der Güte (Abstand der Stützstellen) des Wirkungsgradkennfeldes.
  EMaschine_Output : Inport
  Fluid_Leistungselektronik_Output : Inport  Port=2
  Getriebe_Output : Inport  Port=3
  T_Umgebung [K] : Inport  Port=4
  v_Fahrzeug [m*s^-1] : Inport  Port=5
  Bus Creator : BusCreator  Inputs=4
  Bus Selector : BusSelector  OutputSignals=T_FinitesVolumen_Leistungselektronik(1) [K],PV_Kuehlfluessigkeit_Leistungselektronik(1) [m^3*s^-1]
  Bus Selector1 : BusSelector  OutputSignals=M_EMaschine [Nm],n_EMaschine [min^-1]
  Bus Selector2 : BusSelector  OutputSignals=P_Leistungselektronik [W]
  Divide : Product  Inputs=/*
  Gain : Gain  Gain=eta_Leistungselektronik_Faktor_Volllast
  Leistungselektronik(1) thermisch : Subsystem
  M_EMaschine_max : Lookup_n-D  NumberOfTableDimensions=1  BreakpointsForDimension1=M_EMaschine_max(1,:)  BeginIndexSearchUsingPreviousIndexResult=on  Table=M_EMaschine_max(2,:)  ExtrapMethod=Clip  UseLastTableValue=on  InternalRulePriority=Speed  RndMeth=Simplest  InputSameDT=on
  Relational Operator : RelationalOperator  Operator=<  OutDataTypeStr=boolean  RndMeth=Simplest
  Subtract : Sum  Inputs=+-
  Switch : Switch  Criteria=u2 > Threshold
  Wirkungsgradkennfeld : Lookup_n-D  BreakpointsForDimension1=eta_Leistungselektronik_Break_M_EMaschine  BreakpointsForDimension2=eta_Leistungselektronik_Break_n_EMaschine  BeginIndexSearchUsingPreviousIndexResult=on  Table=eta_Leistungselektronik_Table  ExtrapMethod=Clip  UseLastTableValue=on  InternalRulePriority=Speed  RndMeth=Simplest  InputSameDT=on
  Leistungselektronik_Output : Outport
  wires:
  Leistungselektronik(1) thermisch/2(PQ_Leistungselektronik_FinitesVolumen [W]) -> Bus Creator/4  "PQ_Leistungselektronik(1)_FinitesVolumen [W]"
  Bus Selector2/1 -> Divide/2, Subtract/2  "<P_Leistungselektronik [W]>"
  Divide/1 -> Subtract/1, Bus Creator/2  "P_Batteriepack_Fahrbetrieb [W]"
  Leistungselektronik(1) thermisch/1(T_Leistungselektronik [K]) -> Bus Creator/3  "T_Leistungselektronik [K]"
  Getriebe_Output/1 -> Bus Selector1/1
  Bus Selector1/1 -> Switch/1, Relational Operator/1  "<M_EMaschine [Nm]>"
  Bus Selector1/2 -> Wirkungsgradkennfeld/2, M_EMaschine_max/1  "<n_EMaschine [min^-1]>"
  Subtract/1 -> Leistungselektronik(1) thermisch/1(P_Verlust_Leistungselektronik [W])  "P_Verlust_Leistungselektronik [W]"
  EMaschine_Output/1 -> Bus Selector2/1
  T_Umgebung [K]/1 -> Leistungselektronik(1) thermisch/4(T_Umgebung [K])
  Relational Operator/1 -> Switch/2
  Switch/1 -> Wirkungsgradkennfeld/1
  M_EMaschine_max/1 -> Gain/1
  Gain/1 -> Switch/3, Relational Operator/2
  Wirkungsgradkennfeld/1 -> Divide/1, Bus Creator/1  "eta_Leistungselektronik [-]"
  v_Fahrzeug [m*s^-1]/1 -> Leistungselektronik(1) thermisch/5(v_Fahrzeug [m*s^-1])
  Fluid_Leistungselektronik_Output/1 -> Bus Selector/1
  Bus Selector/2 -> Leistungselektronik(1) thermisch/3(PV_Kuehlfluessigkeit [m^3*s^-1])  "<PV_Kuehlfluessigkeit_Leistungselektronik(1) [m^3*s^-1]>"
  Bus Selector/1 -> Leistungselektronik(1) thermisch/2(T_FinitesVolumen [K])  "<T_FinitesVolumen_Leistungselektronik(1) [K]>"
  Bus Creator/1 -> Leistungselektronik_Output/1

== system mod_sim_VTMS/Thermomanagementsystem/PCM ==
  note: -> Der PCM Speicher funktioniert als thermische Masse.
      | -> Es fällt keine Verlustleistung an.
      | -> Phasenwechselmaterialien ermöglichen über die chemische Zusammensetzung, dass der Phasenwechsel z.B. zwischen fest und flüssig bei einer gewünschten Temperatur stattfinden.
      | -> Der entscheidende Aspekt ist dabei, dass für diesen Phasenwechsel Energie in Form der Schmelz- und Erstarrungsenthalpie an den Phasengrenzen benötigt wird. Dabei bleibt die Temperatur nahezu konstant und es ist möglich das Temperaturniveau von Komponenten im optimalen Betriebsbereich zu halten
      | -> Mit diesem Simulationsmodell kommen zwei Arten von PCM modelliert werden:
      | - PCM, die bei Temperaturerhöhung im Phasenübergang latente Wärme speichern und während des Abkühlens und bei der Rückwandlung wieder abgeben
      | - PCM mit der Charakteristik der unterkühlten Schmelze, die nach vollendeter Umwandlung die Wärme über längere Zeit speichern und gezielt bei Bedarf wieder abgeben können
  Fluid_PCM_Output : Inport
  T_Umgebung [K] : Inport  Port=2
  v_Fahrzeug [m*s^-1] : Inport  Port=3
  Bus Creator : BusCreator  Inputs=4
  Bus Selector : BusSelector  OutputSignals=T_FinitesVolumen_PCM(1) [K],PV_Kuehlfluessigkeit_PCM(1) [m^3*s^-1],T_FinitesVolumen_PCM(2) [K],PV_Kuehlfluessigkeit_PCM(2) [m^3*s^-1]
  PCM thermisch : Subsystem
  PCM_Output : Outport
  wires:
  Bus Creator/1 -> PCM_Output/1
  Fluid_PCM_Output/1 -> Bus Selector/1

== system mod_sim_VTMS/Thermomanagementsystem/Peltier ==
  note: Das Peltier-Element ist eine thermoelektrische Wärmepumpe, die den Kühlkreislauf sowohl vorwärmen als auch kühlen kann.
      | Über ein Steuerungssignal kann das Peltier-Element aktiviert werden
      | Die notwendige elektrische Leistung wird aus der Traktionsbatterie entnommen
      | Die tatsächliche Wärme- und Kühlleistung wird im Block Wirkungsgradbestimmung abhängig von der Kühlwasser- und Umgebungstemperatur bestimmt.
      | Die Umwandlung der Leistung in einen Wärmestrom wird im Block "Peltier thermisch" durchgeführt.
  Fluid_Peltier_Output : Inport
  T_Umgebung : Inport  Port=2
  Abs : Abs
  Bus Creator : BusCreator  Inputs=3
  Bus Selector : BusSelector  OutputSignals=T_FinitesVolumen_Peltier(1) [K]
  From Workspace : FromWorkspace  VariableName=Steuerung_Peltier  SampleTime=0  OutputAfterFinalValue=Setting to zero
  Peltier(1) elektrisch : Subsystem
  Peltier(1) thermisch : Subsystem
  Peltier_Output : Outport
  wires:
  Bus Creator/1 -> Peltier_Output/1
  Peltier(1) thermisch/1(PQ_Peltier_FinitesVolumen [W]) -> Bus Creator/3  "PQ_Peltier(1)_FinitesVolumen [W]"
  Fluid_Peltier_Output/1 -> Bus Selector/1
  Bus Selector/1 -> Peltier(1) elektrisch/3(T_Fluidvolumen_Peltier), Peltier(1) thermisch/2(T_FinitesVolumen [K])  "<T_FinitesVolumen_Peltier(1) [K]>"
  T_Umgebung/1 -> Peltier(1) elektrisch/1(T_Umgebung)
  Peltier(1) elektrisch/1("P_el ") -> Bus Creator/1  "P_Peltier_Bat [W]"
  Peltier(1) elektrisch/2(PQ) -> Bus Creator/2, Peltier(1) thermisch/1(P_Peltier [W])  "PQ_ges"
  From Workspace/1 -> Abs/1, Peltier(1) elektrisch/2(Waermen_Kuehlen)
  Abs/1 -> Peltier(1) elektrisch/Enable

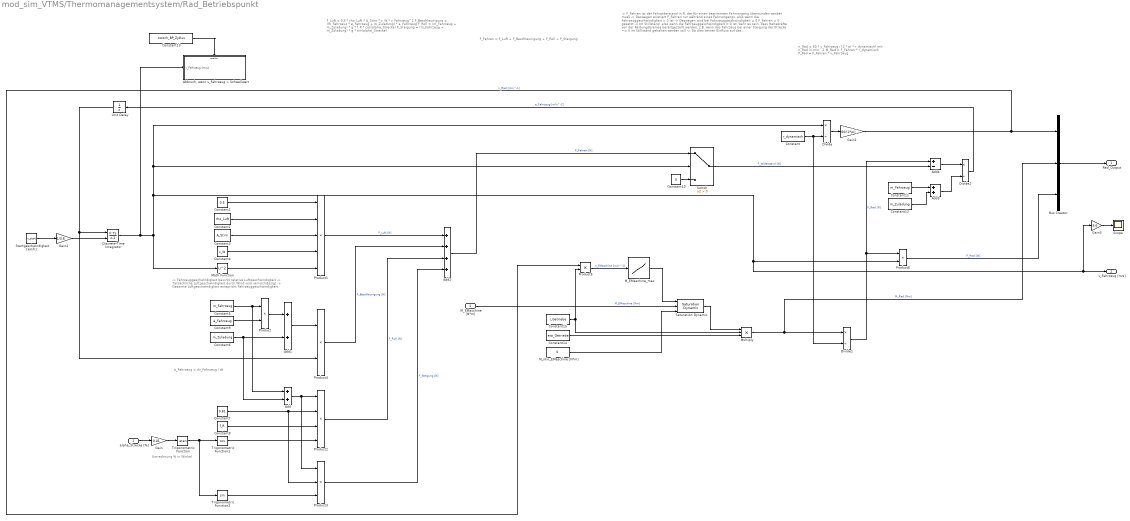
== system mod_sim_VTMS/Thermomanagementsystem/Rad_Betriebspunkt ==
  note: -> F_Fahren ist der Fahrwiderstand in N, der für einen bestimmten Fahrvorgang überwunden werden muss
      | -> Deswegen existiert F_Fahren nur während eines Fahrvorgangs, also wenn die Fahrzeuggeschwindigkeit > 0 ist
      | -> Deswegen wird bei Fahrzeuggeschwindigkeit = 0 F_Fahren = 0 gesetzt
      |
      | -> Im Stillstand, also wenn die Fahrzeuggeschwindigkeit = 0 ist, kann es sein, dass Haltekräfte von der Reibungsbremse bereitgestellt werden, z.B. wenn das Fahrzeug bei einer Steigung der Strecke ~= 0 im Stillstand gehalten werden soll
      | -> Da dies keinen Einfluss auf das Thermomanagementsystemsystem eines Fahrzeugs hat, werden mögliche Haltekräfte im Thermomanagementsystemmodell nicht betrachtet
      | -> Da das Drehmoment der Räder und die Leistungsanforderung an die Räder nur abh. von F_Fahren berechnet werden, werden an den Rädern nur Drehmomente und Leistungsanforderungen aus dem Fahrbetrieb betrachtet, nicht jedoch aus dem Stillstandsbetrieb
  note: n_Rad = 60 * v_Fahrzeug / (2 * pi * r_dynamisch)
      | mit n_Rad in min^-1
      |
      | M_Rad = F_Fahren * r_dynamisch
      |
      | P_Rad = F_Fahren * v_Fahrzeug
  note: F_Luft = 0.5 * rho_Luft * A_Stirn * c_W * v_Fahrzeug^2
      |
      | F_Beschleunigung = (m_Fahrzeug * e_Fahrzeug + m_Zuladung) * a_Fahrzeug
      |
      | F_Roll = (m_Fahrzeug + m_Zuladung) * g * f_R * cos(alpha_Strecke)
      |
      | F_Steigung = (m_Fahrzeug + m_Zuladung) * g * sin(alpha_Strecke)
  note: F_Fahren = F_Luft + F_Beschleunigung + F_Roll + F_Steigung
  note: -> Fahrzeuggeschwindigkeit bewirkt relative Luftgeschwindigkeit
      | -> Tatsächliche Luftgeschwindigkeit durch Wind wird vernachlässigt
      | -> Gesamte Luftgeschwindigkeit entspricht Fahrzeuggeschwindigkeit
  note: a_Fahrzeug = dv_Fahrzeug / dt
  note: Umrechnung % in Winkel
  alpha_Strecke [%] : Inport
  M_EMaschine [N*m] : Inport  Port=2
  "Abbruch, wenn v_Fahrzeug > Schwellwert" : Subsystem
  Add : Sum
  Add1 : Sum
  Add2 : Sum  Inputs=4
  Add3 : Sum
  Add4 : Sum  Inputs=+-
  Bus Creator : BusCreator  Inputs=3
  Constant : Constant  Value=r_dynamisch  VectorParams1D=off
  Constant1 : Constant  Value=0.5  VectorParams1D=off
  Constant10 : Constant  Value=0  VectorParams1D=off
  Constant11 : Constant  Value=m_Fahrzeug  VectorParams1D=off
  Constant12 : Constant  Value=m_Zuladung  VectorParams1D=off
  Constant13 : Constant  Value=switch_BP_Zyklus
  Constant14 : Constant  Value=eta_Getriebe
  Constant15 : Constant  Value=i_Getriebe
  Constant2 : Constant  Value=rho_Luft  VectorParams1D=off
  Constant3 : Constant  Value=A_Stirn  VectorParams1D=off
  Constant4 : Constant  Value=c_W  VectorParams1D=off
  Constant5 : Constant  Value=m_Fahrzeug  VectorParams1D=off
  Constant6 : Constant  Value=m_Zuladung  VectorParams1D=off
  Constant7 : Constant  Value=9.81  VectorParams1D=off
  Constant8 : Constant  Value=f_R  VectorParams1D=off
  Constant9 : Constant  Value=e_Fahrzeug  VectorParams1D=off
  Discrete-Time Integrator : DiscreteIntegrator  InitialConditionSource=external  SampleTime=-1  ICPrevOutput=DiscIntNeverNeededParam  ICPrevScaledInput=DiscIntNeverNeededParam
  Divide : Product  Inputs=*/
  Divide1 : Product  Inputs=*/
  Divide2 : Product  Inputs=*/
  Gain : Gain  Gain=0.01
  Gain1 : Gain  Gain=60/(2*pi)
  Gain2 : Gain  Gain=1/3.6
  Gain3 : Gain  Gain=3.6
  M_EMaschine_max : Lookup_n-D  NumberOfTableDimensions=1  BreakpointsForDimension1=M_EMaschine_max(1,:)  BeginIndexSearchUsingPreviousIndexResult=on  Table=M_EMaschine_max(2,:)  ExtrapMethod=Clip  UseLastTableValue=on  InternalRulePriority=Speed  RndMeth=Simplest  InputSameDT=on
  M_min_EMaschine [N*m] : Constant  Value=0
  Math Function : Math  Operator=square  SaturateOnIntegerOverflow=on
  Multiply : Product  Inputs=3
  Product{,4..6} (4 alike) : Product
  Product1 : Product  Inputs=5
  Product2 : Product  Inputs=4
  Product3 : Product  Inputs=3
  Saturation Dynamic : simulink/Discontinuities/Saturation Dynamic  OutMin=[]  OutMax=[]  OutDataTypeStr=Inherit: Same as second input  OutDataType=fixdt(1, 16)  OutScaling=2^-10  DoSatur=off
  Scope : Scope
  "Startgeschwindigkeit [km/h] " : Constant  Value=v_start
  Switch : Switch  Criteria=u2 > Threshold
  Trigonometric Function : Trigonometry  Operator=atan
  Trigonometric Function1 : Trigonometry  Operator=cos
  Trigonometric Function2 : Trigonometry
  Unit Delay : UnitDelay  SampleTime=-1
  Rad_Output : Outport
  v_Fahrzeug [m/s] : Outport  Port=2
  wires:
  Product6/1 -> Bus Creator/3  "P_Rad [W]"
  Constant5/1 -> Add/1, Product/1
  Constant6/1 -> Add1/2, Add/2
  Constant9/1 -> Product/2
  Product/1 -> Add1/1
  Divide2/1 -> Unit Delay/1  "a_Fahrzeug [m*s^-2]"
  Add1/1 -> Product4/1
  Product1/1 -> Add2/1  "F_Luft [N]"
  Product4/1 -> Add2/2  "F_Beschleunigung [N]"
  Trigonometric Function/1 -> Trigonometric Function2/1, Trigonometric Function1/1
  Add/1 -> Product3/1, Product2/1
  Constant7/1 -> Product3/2, Product2/2
  Trigonometric Function2/1 -> Product3/3
  Product3/1 -> Add2/4  "F_Steigung [N]"
  Trigonometric Function1/1 -> Product2/4
  Constant8/1 -> Product2/3
  Product2/1 -> Add2/3  "F_Roll [N]"
  alpha_Strecke [%]/1 -> Gain/1
  Gain/1 -> Trigonometric Function/1
  Constant/1 -> Divide/2, Divide1/2
  Divide/1 -> Gain1/1
  M_EMaschine [N*m]/1 -> Saturation Dynamic/2  "M_EMaschine [Nm]"
  Gain1/1 -> Bus Creator/1, Product5/1  "n_Rad [min^-1]"
  Bus Creator/1 -> Rad_Output/1
  Constant3/1 -> Product1/3
  Constant1/1 -> Product1/1
  Constant2/1 -> Product1/2
  Constant4/1 -> Product1/4
  Math Function/1 -> Product1/5
  Add2/1 -> Switch/1  "F_Fahren [N]"
  Constant10/1 -> Switch/3
  Switch/1 -> Add4/2  "F_Widerstand [N]"
  Constant11/1 -> Add3/1
  Constant12/1 -> Add3/2
  Divide1/1 -> Add4/1, Product6/1  "F_Rad [N]"
  Add4/1 -> Divide2/1
  Add3/1 -> Divide2/2
  Discrete-Time Integrator/1 -> "Abbruch, wenn v_Fahrzeug > Schwellwert"/1(v_Fahrzeug [m/s]), Math Function/1, Product6/2, Gain3/1, v_Fahrzeug [m/s]/1, Switch/2, Divide/1
  "Startgeschwindigkeit [km/h] "/1 -> Gain2/1
  Gain2/1 -> Discrete-Time Integrator/2
  Unit Delay/1 -> Product4/2, Discrete-Time Integrator/1
  Saturation Dynamic/1 -> Multiply/1
  M_min_EMaschine [N*m]/1 -> Saturation Dynamic/3
  M_EMaschine_max/1 -> Saturation Dynamic/1
  Product5/1 -> M_EMaschine_max/1  "n_EMaschine [min^-1]"
  Constant14/1 -> Multiply/3
  Multiply/1 -> Bus Creator/2, Divide1/1  "M_Rad [Nm]"
  Constant15/1 -> Multiply/2, Product5/2
  Gain3/1 -> Scope/1
  Constant13/1 -> "Abbruch, wenn v_Fahrzeug > Schwellwert"/Enable

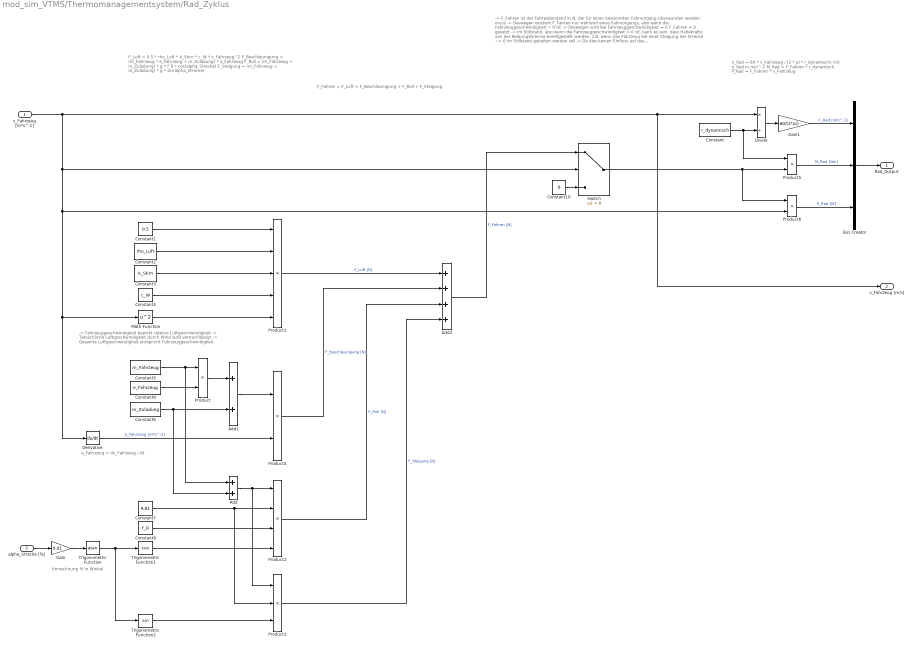
== system mod_sim_VTMS/Thermomanagementsystem/Rad_Zyklus ==
  note: -> F_Fahren ist der Fahrwiderstand in N, der für einen bestimmten Fahrvorgang überwunden werden muss
      | -> Deswegen existiert F_Fahren nur während eines Fahrvorgangs, also wenn die Fahrzeuggeschwindigkeit > 0 ist
      | -> Deswegen wird bei Fahrzeuggeschwindigkeit = 0 F_Fahren = 0 gesetzt
      |
      | -> Im Stillstand, also wenn die Fahrzeuggeschwindigkeit = 0 ist, kann es sein, dass Haltekräfte von der Reibungsbremse bereitgestellt werden, z.B. wenn das Fahrzeug bei einer Steigung der Strecke ~= 0 im Stillstand gehalten werden soll
      | -> Da dies keinen Einfluss auf das Thermomanagementsystemsystem eines Fahrzeugs hat, werden mögliche Haltekräfte im Thermomanagementsystemmodell nicht betrachtet
      | -> Da das Drehmoment der Räder und die Leistungsanforderung an die Räder nur abh. von F_Fahren berechnet werden, werden an den Rädern nur Drehmomente und Leistungsanforderungen aus dem Fahrbetrieb betrachtet, nicht jedoch aus dem Stillstandsbetrieb
  note: n_Rad = 60 * v_Fahrzeug / (2 * pi * r_dynamisch)
      | mit n_Rad in min^-1
      |
      | M_Rad = F_Fahren * r_dynamisch
      |
      | P_Rad = F_Fahren * v_Fahrzeug
  note: F_Luft = 0.5 * rho_Luft * A_Stirn * c_W * v_Fahrzeug^2
      |
      | F_Beschleunigung = (m_Fahrzeug * e_Fahrzeug + m_Zuladung) * a_Fahrzeug
      |
      | F_Roll = (m_Fahrzeug + m_Zuladung) * g * f_R * cos(alpha_Strecke)
      |
      | F_Steigung = (m_Fahrzeug + m_Zuladung) * g * sin(alpha_Strecke)
  note: F_Fahren = F_Luft + F_Beschleunigung + F_Roll + F_Steigung
  note: -> Fahrzeuggeschwindigkeit bewirkt relative Luftgeschwindigkeit
      | -> Tatsächliche Luftgeschwindigkeit durch Wind wird vernachlässigt
      | -> Gesamte Luftgeschwindigkeit entspricht Fahrzeuggeschwindigkeit
  note: a_Fahrzeug = dv_Fahrzeug / dt
  note: Umrechnung % in Winkel
  v_Fahrzeug [m*s^-1] : Inport
  alpha_Strecke [%] : Inport  Port=2
  Add : Sum
  Add1 : Sum
  Add2 : Sum  Inputs=4
  Bus Creator : BusCreator  Inputs=3
  Constant : Constant  Value=r_dynamisch  VectorParams1D=off
  Constant1 : Constant  Value=0.5  VectorParams1D=off
  Constant10 : Constant  Value=0  VectorParams1D=off
  Constant2 : Constant  Value=rho_Luft  VectorParams1D=off
  Constant3 : Constant  Value=A_Stirn  VectorParams1D=off
  Constant4 : Constant  Value=c_W  VectorParams1D=off
  Constant5 : Constant  Value=m_Fahrzeug  VectorParams1D=off
  Constant6 : Constant  Value=m_Zuladung  VectorParams1D=off
  Constant7 : Constant  Value=9.81  VectorParams1D=off
  Constant8 : Constant  Value=f_R  VectorParams1D=off
  Constant9 : Constant  Value=e_Fahrzeug  VectorParams1D=off
  Derivative : Derivative
  Divide : Product  Inputs=*/
  Gain : Gain  Gain=0.01
  Gain1 : Gain  Gain=60/(2*pi)
  Math Function : Math  Operator=square  SaturateOnIntegerOverflow=on
  Product{,4..6} (4 alike) : Product
  Product1 : Product  Inputs=5
  Product2 : Product  Inputs=4
  Product3 : Product  Inputs=3
  Switch : Switch  Criteria=u2 > Threshold
  Trigonometric Function : Trigonometry  Operator=atan
  Trigonometric Function1 : Trigonometry  Operator=cos
  Trigonometric Function2 : Trigonometry
  Rad_Output : Outport
  v_Fahrzeug [m/s] : Outport  Port=2
  wires:
  v_Fahrzeug [m*s^-1]/1 -> v_Fahrzeug [m/s]/1, Divide/1, Product6/2, Math Function/1, Derivative/1, Switch/2
  Product6/1 -> Bus Creator/3  "P_Rad [W]"
  Constant5/1 -> Add/1, Product/1
  Constant6/1 -> Add1/2, Add/2
  Constant9/1 -> Product/2
  Product/1 -> Add1/1
  Derivative/1 -> Product4/2  "a_Fahrzeug [m*s^-2]"
  Add1/1 -> Product4/1
  Product1/1 -> Add2/1  "F_Luft [N]"
  Product4/1 -> Add2/2  "F_Beschleunigung [N]"
  Trigonometric Function/1 -> Trigonometric Function2/1, Trigonometric Function1/1
  Add/1 -> Product3/1, Product2/1
  Constant7/1 -> Product3/2, Product2/2
  Trigonometric Function2/1 -> Product3/3
  Product3/1 -> Add2/4  "F_Steigung [N]"
  Trigonometric Function1/1 -> Product2/4
  Constant8/1 -> Product2/3
  Product2/1 -> Add2/3  "F_Roll [N]"
  alpha_Strecke [%]/1 -> Gain/1
  Gain/1 -> Trigonometric Function/1
  Constant/1 -> Divide/2, Product5/1
  Divide/1 -> Gain1/1
  Product5/1 -> Bus Creator/2  "M_Rad [Nm]"
  Gain1/1 -> Bus Creator/1  "n_Rad [min^-1]"
  Bus Creator/1 -> Rad_Output/1
  Constant3/1 -> Product1/3
  Constant1/1 -> Product1/1
  Constant2/1 -> Product1/2
  Constant4/1 -> Product1/4
  Math Function/1 -> Product1/5
  Add2/1 -> Switch/1  "F_Fahren [N]"
  Constant10/1 -> Switch/3
  Switch/1 -> Product5/2, Product6/1
